simulink model "quadcopter_model_HITL"  (R2022b)
settings: Solver=FixedStepAuto  StartTime=0.0  StopTime=10.0  RelTol=1e-3
values from neighbouring files (symbols this model uses):
  g = 9.81    [load_model_parameters.m]
  Ix = 2.353 * exp(-3)    [load_model_parameters.m]
  Iy = 2.353 * exp(-3)    [load_model_parameters.m]
  Iz = 5.262 * exp(-2)    [load_model_parameters.m]
  m = 1.2    [load_model_parameters.m]
settings Model: Creator=paolo  LastModifiedBy=paolo

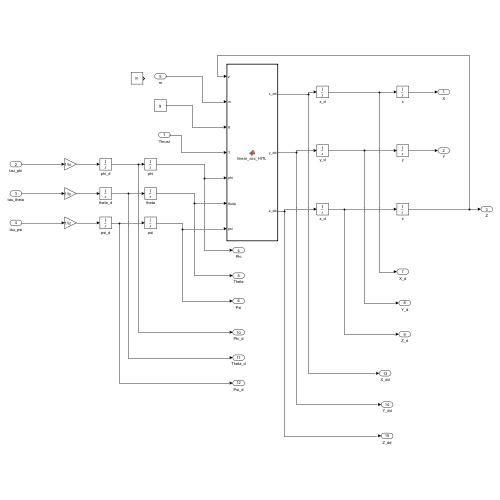
[thumbnail: Simulink's stored preview of the top-level diagram]
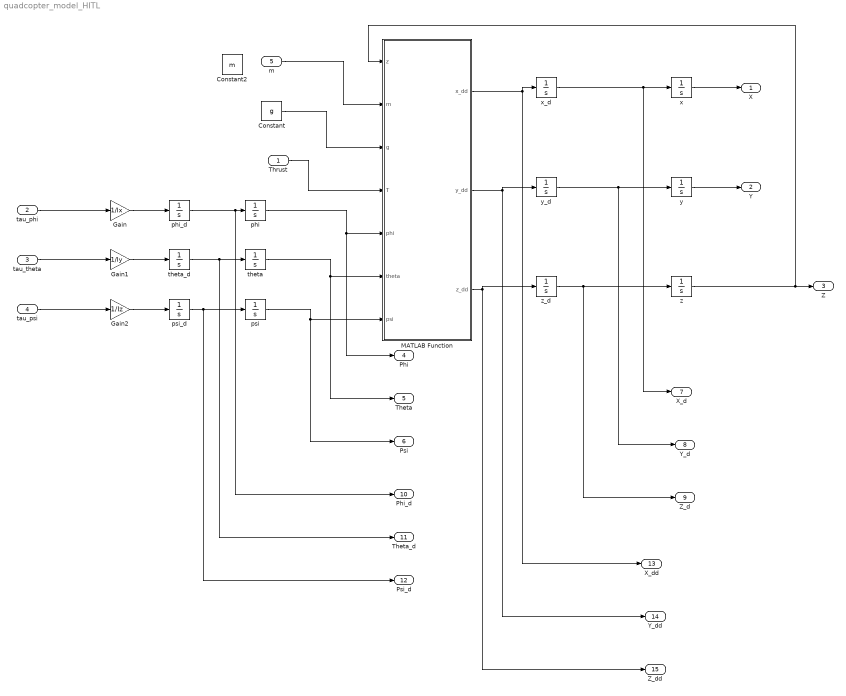
== system quadcopter_model_HITL ==
  Thrust : Inport
  tau_phi : Inport  Port=2
  tau_theta : Inport  Port=3
  tau_psi : Inport  Port=4
  m : Inport  Port=5
  Constant : Constant  Value=g
  Constant2 : Constant  Value=m
  Gain : Gain  Gain=1/Ix
  Gain1 : Gain  Gain=1/Iy
  Gain2 : Gain  Gain=1/Iz
  MATLAB Function : MATLAB Function  TreatAsAtomicUnit=on
  phi : Integrator
  phi_d : Integrator
  psi : Integrator
  psi_d : Integrator
  theta : Integrator
  theta_d : Integrator
  x : Integrator
  x_d : Integrator
  y : Integrator  InitialCondition=0.01
  y_d : Integrator
  z : Integrator  UpperSaturationLimit=0
  z_d : Integrator  UpperSaturationLimit=0
  X : Outport
  Y : Outport  Port=2
  Z : Outport  Port=3
  Phi : Outport  Port=4
  Theta : Outport  Port=5
  Psi : Outport  Port=6
  X_d : Outport  Port=7
  Y_d : Outport  Port=8
  Z_d : Outport  Port=9
  Phi_d : Outport  Port=10
  Theta_d : Outport  Port=11
  Psi_d : Outport  Port=12
  X_dd : Outport  Port=13
  Y_dd : Outport  Port=14
  Z_dd : Outport  Port=15
  wires:
  tau_phi/1 -> Gain/1
  tau_theta/1 -> Gain1/1
  tau_psi/1 -> Gain2/1
  psi/1 -> Psi/1, MATLAB Function/7(psi)
  theta/1 -> Theta/1, MATLAB Function/6(theta)
  phi/1 -> Phi/1, MATLAB Function/5(phi)
  Thrust/1 -> MATLAB Function/4(T)
  m/1 -> MATLAB Function/2(m)
  y/1 -> Y/1
  x/1 -> X/1
  x_d/1 -> X_d/1, x/1
  y_d/1 -> Y_d/1, y/1
  z_d/1 -> z/1, Z_d/1
  psi_d/1 -> psi/1, Psi_d/1
  theta_d/1 -> theta/1, Theta_d/1
  phi_d/1 -> Phi_d/1, phi/1
  Gain/1 -> phi_d/1
  Gain1/1 -> theta_d/1
  Gain2/1 -> psi_d/1
  MATLAB Function/3(z_dd) -> Z_dd/1, z_d/1
  MATLAB Function/1(x_dd) -> X_dd/1, x_d/1
  MATLAB Function/2(y_dd) -> Y_dd/1, y_d/1
  z/1 -> MATLAB Function/1(z), Z/1
  Constant/1 -> MATLAB Function/3(g)

== matlab function quadcopter_model_HITL/MATLAB Function ==
  data: z input; m input; x_dd output; g input; T input; phi input; theta input; psi input; y_dd output; z_dd output
 function [x_dd, y_dd, z_dd] = linear_acc_HITL(z, m, g, T, phi, theta, psi)

x_dd = -(cos(psi)*sin(theta)*cos(phi) + sin(psi)*sin(phi)) * (T/m);
y_dd = -(sin(psi)*sin(theta)*cos(phi) - sin(phi)*cos(psi)) * (T/m);
z_dd = -(cos(theta)*cos(phi)*(T/m)) + g;

if z >= 0 && z_dd > 0
    z_dd = 0;

end
